simulink model "lin_model_PI_MRAC_Sim_CASE2_v2"  (Simulink 7.7)
settings: Solver=ode45  StartTime=0.0  StopTime=TIME  RelTol=1e-3  AbsTol=1e-6
values from neighbouring files (symbols this model uses):
  AA = A_cruise    [parameter.m]
  Am = AA - BB*Kr    [lin_model_LQR.m]    (also in lin_model_PI_MRAC_CASE1.m = Ar-BB*Kr; lin_model_PI_MRAC_CASE1_L1.m = Ar-BB*Kr)
  BB = B_cruise    [parameter.m]
  theta_hat0 = eye(11)    [lin_model_PI_MRAC_CASE1.m]    (also in lin_model_PI_MRAC_CASE1_L1.m)
  x0 = [0;0;0;0]    [beta_crS.m]    (also in flapping.m = []; flappingthrust.m = []; lin_flapping.m = []; lin_model_LQR.m = [3 3 3 0 0 0 0 0 0 0 0]')
  x_hat0 = x0    [lin_model_PI_MRAC_CASE1.m]    (also in lin_model_PI_MRAC_CASE1_L1.m)
undefined symbols (not defined in the file or in its folder): Br, gamma1, gamma2, kg, Kr, Theta_b_hat0
libraries: dspmtrx3 x2, dspinverses x1, simulink x1
settings Model: Creator=Li  LastModifiedBy=Li
settings DataIOCC: LimitDataPoints=off  SaveFormat=StructureWithTime
settings DebuggingCC: SolverPrmCheckMsg=none

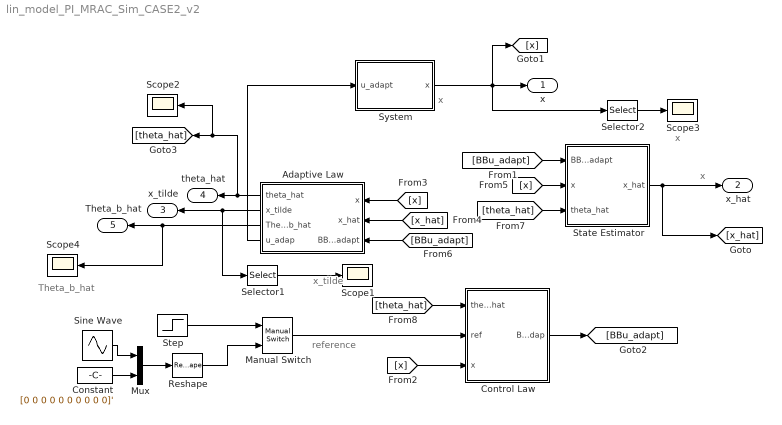
== system lin_model_PI_MRAC_Sim_CASE2_v2 ==
  note: x
  note: reference
  note: Theta_b_hat
  note: x_tilde
  note: x
  note: x
  Adaptive Law : Subsystem
  Constant : Constant  Value=[0 0 0 0 0 0 0 0 0 0]'
  Control Law : Subsystem
  Manual Switch : simulink/Signal Routing/Manual Switch  SystemSampleTime=-1  sw=1  action=0  varsize=off
  Mux : Mux  Inputs=2
  Reshape : Reshape  OutputDimensionality=Column vector (2-D)
  Scope{1..4} (4 alike) : Scope
      Scope1 settings: TimeRange=3  YMin=-0.4  YMax=2
      Scope2 settings: TimeRange=5  YMin=-75  YMax=25
      Scope3 settings: TimeRange=5  YMin=-0.014  YMax=0.001  SaveName=ScopeData2
      Scope4 settings: TimeRange=5  YMin=-3.5  YMax=3  SaveName=ScopeData3
  Selector1 : Selector  InputPortWidth=11  IndexOptions=Index vector (dialog)  Indices=[1 2 3 4 5]  OutputSizes=1
  Selector2 : Selector  InputPortWidth=11  IndexOptions=Index vector (dialog)  Indices=[1 2 3 4 5]  OutputSizes=1
  Sine Wave : Sin  Amplitude=4  Frequency=2  SampleTime=0
  State Estimator : Subsystem
  Step : Step  Time=0  After=[1 -1 2 0 0 0 0 0 0 0 0]'  SampleTime=0
  System : Subsystem
  x : Outport
  x_hat : Outport  Port=2
  x_tilde : Outport  Port=3
  theta_hat : Outport  Port=4
  Theta_b_hat : Outport  Port=5
  wires:
  State Estimator/1(x_hat) -> x_hat/1, [x_hat]
  [BBu_adapt] -> State Estimator/1(BBu_adapt)
  Control Law/1(BBu_adap) -> [BBu_adapt]
  Step/1 -> Manual Switch/1
  Manual Switch/1 -> Control Law/2(ref)
  Sine Wave/1 -> Mux/1
  Constant/1 -> Mux/2
  Mux/1 -> Reshape/1
  Reshape/1 -> Manual Switch/2
  Selector1/1 -> Scope1/1
  Selector2/1 -> Scope3/1
  [x] -> Control Law/3(x)
  [x] -> State Estimator/2(x)
  [theta_hat] -> State Estimator/3(theta_hat)
  [theta_hat] -> Control Law/1(theta_hat)
  [BBu_adapt] -> Adaptive Law/3(BBu_adapt)
  [x_hat] -> Adaptive Law/2(x_hat)
  [x] -> Adaptive Law/1(x)
  Adaptive Law/1(theta_hat) -> theta_hat/1, [theta_hat], Scope2/1
  Adaptive Law/2(x_tilde) -> x_tilde/1, Selector1/1
  Adaptive Law/3(Theta_b_hat) -> Theta_b_hat/1, Scope4/1
  System/1(x) -> x/1, Selector2/1, [x]
  Adaptive Law/4(u_adap) -> System/1(u_adapt)

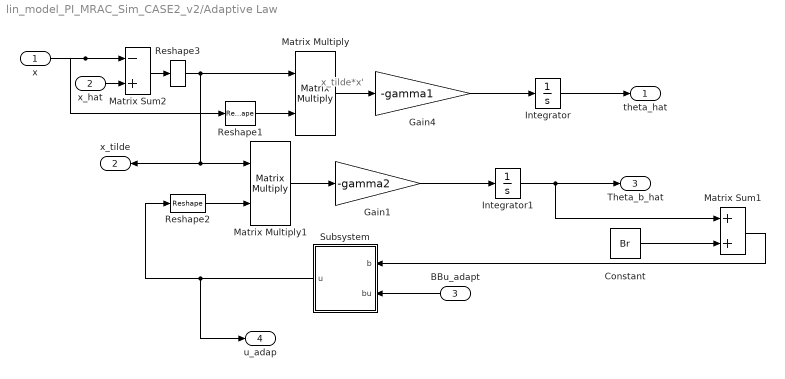
== system lin_model_PI_MRAC_Sim_CASE2_v2/Adaptive Law ==
  note: x_tilde*x'
  x : Inport
  x_hat : Inport  Port=2
  BBu_adapt : Inport  Port=3
  Constant : Constant  Value=Br
  Gain1 : Gain  Gain=-gamma2
  Gain4 : Gain  Gain=-gamma1
  Integrator : Integrator  InitialCondition=theta_hat0
  Integrator1 : Integrator  InitialCondition=Theta_b_hat0
  Matrix Sum1 : Sum
  Matrix Sum2 : Sum  Inputs=-+
  Matrix Multiply : Product  Multiplication=Matrix(*)
  Matrix Multiply1 : Product  Multiplication=Matrix(*)
  Reshape1 : Reshape  OutputDimensionality=Row vector (2-D)
  Reshape2 : Reshape  OutputDimensionality=Row vector (2-D)
  Reshape3 : Reshape  OutputDimensionality=Column vector (2-D)
  Subsystem : Subsystem
  theta_hat : Outport
  x_tilde : Outport  Port=2
  Theta_b_hat : Outport  Port=3
  u_adap : Outport  Port=4
  wires:
  Reshape1/1 -> Matrix Multiply/2
  Matrix Multiply/1 -> Gain4/1
  x/1 -> Matrix Sum2/1, Reshape1/1
  x_hat/1 -> Matrix Sum2/2
  Gain4/1 -> Integrator/1
  Integrator/1 -> theta_hat/1
  Gain1/1 -> Integrator1/1
  Matrix Multiply1/1 -> Gain1/1
  Reshape2/1 -> Matrix Multiply1/2
  Matrix Sum2/1 -> Reshape3/1
  Reshape3/1 -> Matrix Multiply/1, Matrix Multiply1/1, x_tilde/1
  Integrator1/1 -> Theta_b_hat/1, Matrix Sum1/1
  Subsystem/1(u) -> Reshape2/1, u_adap/1
  BBu_adapt/1 -> Subsystem/2(bu)
  Constant/1 -> Matrix Sum1/2
  Matrix Sum1/1 -> Subsystem/1(b)

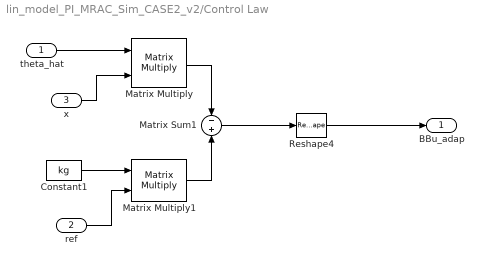
== system lin_model_PI_MRAC_Sim_CASE2_v2/Control Law ==
  theta_hat : Inport
  ref : Inport  Port=2
  x : Inport  Port=3
  Constant1 : Constant  Value=kg
  Matrix Sum1 : Sum  Inputs=-+
  Matrix Multiply : Product  Multiplication=Matrix(*)
  Matrix Multiply1 : Product  Multiplication=Matrix(*)
  Reshape4 : Reshape  OutputDimensionality=Column vector (2-D)
  BBu_adap : Outport
  wires:
  Matrix Multiply/1 -> Matrix Sum1/1
  x/1 -> Matrix Multiply/2
  ref/1 -> Matrix Multiply1/2
  Matrix Multiply1/1 -> Matrix Sum1/2
  Matrix Sum1/1 -> Reshape4/1
  Constant1/1 -> Matrix Multiply1/1
  theta_hat/1 -> Matrix Multiply/1
  Reshape4/1 -> BBu_adap/1

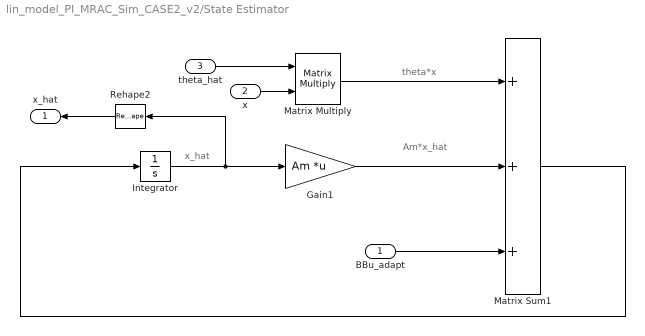
== system lin_model_PI_MRAC_Sim_CASE2_v2/State Estimator ==
  note: x_hat
  note: theta*x
  note: Am*x_hat
  BBu_adapt : Inport
  x : Inport  Port=2
  theta_hat : Inport  Port=3
  Gain1 : Gain  Gain=Am  Multiplication=Matrix(K*u) (u vector)
  Integrator : Integrator  InitialCondition=x_hat0
  Matrix Sum1 : Sum  Inputs=+++
  Matrix Multiply : Product  Multiplication=Matrix(*)
  Rehape2 : Reshape  OutputDimensionality=Column vector (2-D)
  x_hat : Outport
  wires:
  theta_hat/1 -> Matrix Multiply/1
  Integrator/1 -> Gain1/1, Rehape2/1
  Matrix Multiply/1 -> Matrix Sum1/1
  Gain1/1 -> Matrix Sum1/2
  x/1 -> Matrix Multiply/2
  Matrix Sum1/1 -> Integrator/1
  Rehape2/1 -> x_hat/1
  BBu_adapt/1 -> Matrix Sum1/3

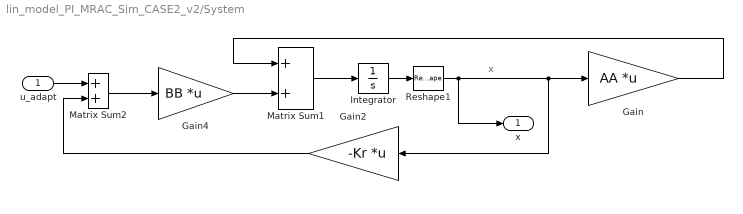
== system lin_model_PI_MRAC_Sim_CASE2_v2/System ==
  note: x
  u_adapt : Inport
  Gain : Gain  Gain=AA  Multiplication=Matrix(K*u) (u vector)
  Gain2 : Gain  Gain=-Kr  Multiplication=Matrix(K*u) (u vector)
  Gain4 : Gain  Gain=BB  Multiplication=Matrix(K*u) (u vector)
  Integrator : Integrator  InitialCondition=x0
  Matrix Sum1 : Sum
  Matrix Sum2 : Sum
  Reshape1 : Reshape  OutputDimensionality=Column vector (2-D)
  x : Outport
  wires:
  Matrix Sum1/1 -> Integrator/1
  Integrator/1 -> Reshape1/1
  Reshape1/1 -> x/1, Gain/1, Gain2/1
  Gain/1 -> Matrix Sum1/1
  Gain4/1 -> Matrix Sum1/2
  u_adapt/1 -> Matrix Sum2/1
  Gain2/1 -> Matrix Sum2/2
  Matrix Sum2/1 -> Gain4/1

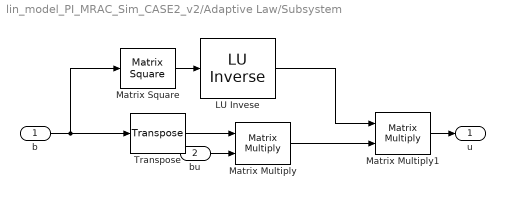
== system lin_model_PI_MRAC_Sim_CASE2_v2/Adaptive Law/Subsystem ==
  b : Inport
  bu : Inport  Port=2
  " LU Invese" : dspinverses/ LU Inverse  SystemSampleTime=-1
  Matrix Square : dspmtrx3/Matrix Square  SystemSampleTime=-1  OutMin=[]  OutMax=[]
  Matrix Multiply : Product  Multiplication=Matrix(*)
  Matrix Multiply1 : Product  Multiplication=Matrix(*)
  Transpose : dspmtrx3/Transpose  SystemSampleTime=-1  Hermitian=off  overflowFlag=off
  u : Outport
  wires:
  b/1 -> Matrix Square/1, Transpose/1
  Transpose/1 -> Matrix Multiply/1
  Matrix Multiply/1 -> Matrix Multiply1/2
  Matrix Square/1 -> " LU Invese"/1
  " LU Invese"/1 -> Matrix Multiply1/1
  Matrix Multiply1/1 -> u/1
  bu/1 -> Matrix Multiply/2
